simulink model "hw01_q03"  (R2024b)
settings: Solver=ode3  StartTime=0.0  StopTime=0.1  FixedStep=0.0001  RelTol=1e-3
undefined symbols (not defined in the file): C_cap, L, r_L
settings Model: Creator=Aryan Ritwajeet Jha  LastModifiedBy=Aryan Ritwajeet Jha

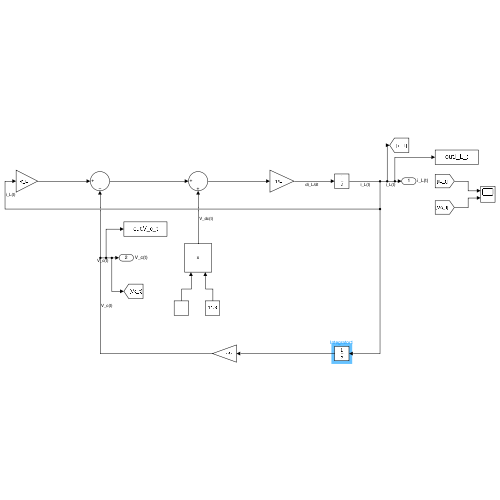
[thumbnail: Simulink's stored preview of the top-level diagram]
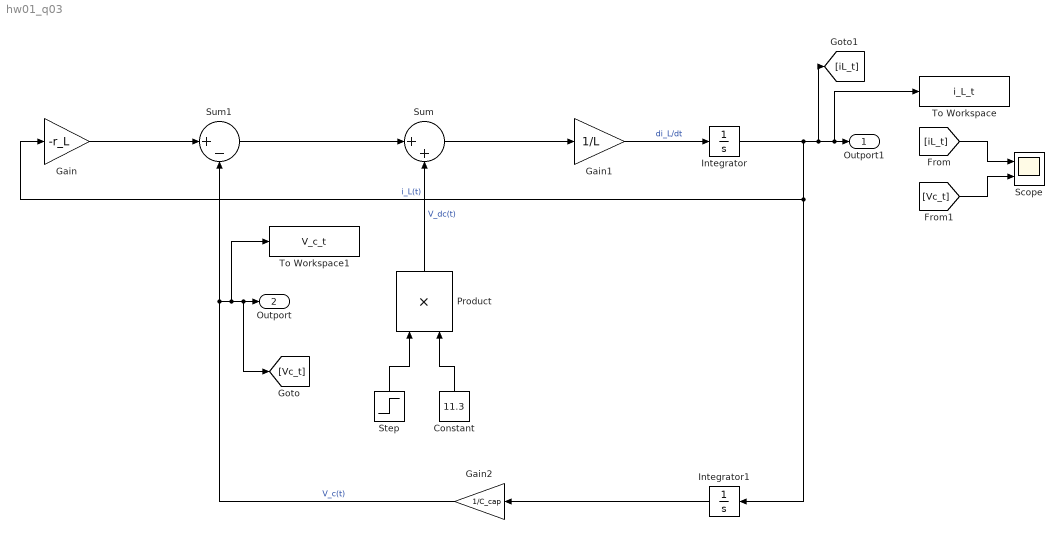
== system hw01_q03 ==
  Constant : Constant  Value=11.3
  Gain : Gain  Gain=-r_L
  Gain1 : Gain  Gain=1/L
  Gain2 : Gain  Gain=1/C_cap
  Integrator : Integrator  ContinuousStateAttributes='i_L_t'
  Integrator1 : Integrator  ContinuousStateAttributes='V_c_t'
  Product : Product
  Scope : Scope  NumInputPorts=2
  Step : Step  Time=0  SampleTime=0
  Sum : Sum  Inputs=|++
  Sum1 : Sum  Inputs=|+-
  To Workspace : ToWorkspace  VariableName=i_L_t  SaveFormat=Timeseries  SampleTime=-1
  To Workspace1 : ToWorkspace  VariableName=V_c_t  SaveFormat=Timeseries  SampleTime=-1
  Outport1 : Outport  SignalName=i_L(t)
  Outport : Outport  Port=2  SignalName=V_c(t)
  wires:
  Step/1 -> Product/1
  Constant/1 -> Product/2
  Product/1 -> Sum/2  "V_dc(t)"
  Sum1/1 -> Sum/1
  Gain/1 -> Sum1/1
  Sum/1 -> Gain1/1
  Gain1/1 -> Integrator/1  "di_L/dt"
  Integrator/1 -> Gain/1, Integrator1/1, [iL_t], To Workspace/1, Outport1/1  "i_L(t)"
  Integrator1/1 -> Gain2/1
  Gain2/1 -> To Workspace1/1, [Vc_t], Outport/1, Sum1/2  "V_c(t)"
  [iL_t] -> Scope/1
  [Vc_t] -> Scope/2
